simulink model "embedded_with_structure"  (Simulink 7.6)
settings: Solver=FixedStepDiscrete  StartTime=0.0  StopTime=10.0  FixedStep=1  RelTol=1e-3
PreLoadFcn:
  | busobjectspec
settings Model: Creator=hnine  LastModifiedBy=c2wt
settings DataIOCC: SaveFormat=Structure
settings OptimizationCC: InitFltsAndDblsToZero=on
settings DebuggingCC: SaveWithParameterizedLinksMsg=none  StrictBusMsg=Warning
settings SFSimCC: SimParseCustomCode=off
settings GRTTargetCC: TargetFcnLib=ansi_tfl_tmw.mat

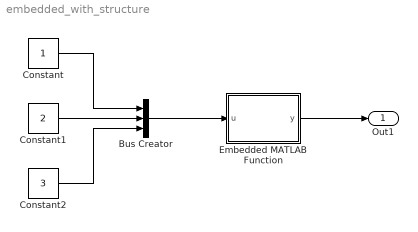
== system embedded_with_structure ==
  Bus Creator : BusCreator  Inputs=3  OutDataTypeStr=Bus: bosecondary  NonVirtualBus=on
  Constant : Constant  OutDataTypeStr=double
  Constant1 : Constant  Value=2  OutDataTypeStr=single
  Constant2 : Constant  Value=3  OutDataTypeStr=uint32
  Embedded MATLAB Function : Stateflow chart  TreatAsAtomicUnit=on
  Out1 : Outport
  wires:
  Constant/1 -> Bus Creator/1
  Constant1/1 -> Bus Creator/2
  Constant2/1 -> Bus Creator/3
  Bus Creator/1 -> Embedded MATLAB Function/1(u)
  Embedded MATLAB Function/1(y) -> Out1/1

== matlab function Embedded MATLAB Function ==
  data: u input Bus: bosecondary; y output double
% SL_CodeGen SHOULD IGNORE LEADING COMMENTS
% ON FUNCTIONS
function y = fcn(u)
%#eml

y = u.Pressure;
